simulink model "radio_enlace"  (R2017a)
settings: Solver=ode45  StartTime=0.0  StopTime=Inf  RelTol=1e-3  EnableMultiTasking=on
libraries: dsparch4 x5, commfilt2 x3, commdigbbndpm3 x2, commsink2 x1, simulink x1, dspstat3 x1, commrflib2 x1, commchan3 x1, commrandsrc2 x1
settings Model: Creator=ampl  LastModifiedBy=rubem
settings DataIOCC: LimitDataPoints=on  SaveFormat=Array
settings OptimizationCC: LifeSpan=inf
settings DebuggingCC: UnderspecifiedInitializationDetection=Classic  MergeDetectMultiDrivingBlocksExec=none  SolverPrmCheckMsg=warning  SFUnexpectedBacktrackingDiag=warning  SFNoUnconditionalDefaultTransitionDiag=warning  SFExecutionAtInitializationDiag=none
settings HardwareCC: ProdBitPerPointer=32  ProdBitPerSizeT=32  ProdBitPerPtrDiffT=32  ProdLargestAtomicFloat=None  ProdIntDivRoundTo=Undefined  ProdEndianess=Unspecified  ProdWordSize=32  ProdHWDeviceType=32-bit Generic
settings ModelReferenceCC: PropagateSignalLabelsOutOfModel=off
settings GRTTargetCC: TargetLangStandard=C89/C90 (ANSI)  GeneratePreprocessorConditionals=Disable all
settings ConfigComp: CovMetricSettings=dw  CovHtmlReporting=on  CovSaveCumulativeToWorkspaceVar=on  CovSaveSingleToWorkspaceVar=on  CovExternalEMLEnable=off

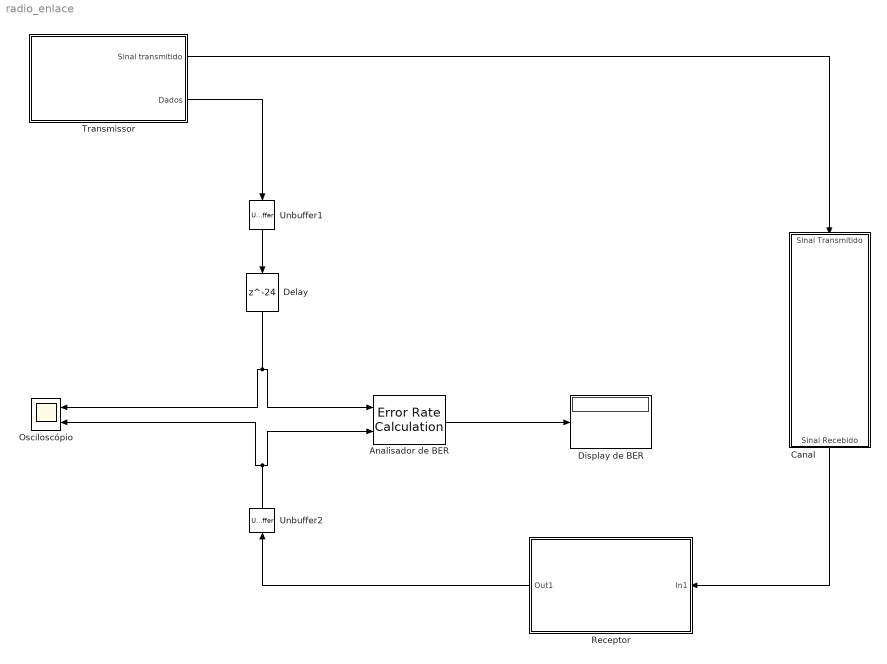
== system radio_enlace ==
  Analisador de BER : commsink2/Error Rate Calculation  N=0  st_delay=1e3  cp_mode=Entire frame  subframe=[]  PMode=Port  WsName=ErrorVec  RsMode2=off  stop=off  numErr=100  maxBits=1e6
  Canal : Subsystem
  Delay : Delay  DelayLength=24
  Display de BER : Display
  Osciloscópio : Scope  NumInputPorts=2
  Receptor : Subsystem
  Transmissor : Subsystem
  Unbuffer1 : Unbuffer
  Unbuffer2 : Unbuffer
  wires:
  Analisador de BER/1 -> Display de BER/1
  Unbuffer1/1 -> Delay/1
  Transmissor/2(Dados) -> Unbuffer1/1
  Transmissor/1(Sinal transmitido) -> Canal/1(Sinal Transmitido)
  Canal/1(Sinal Recebido) -> Receptor/1(In1)
  Receptor/1(Out1) -> Unbuffer2/1
  Unbuffer2/1 -> Osciloscópio/2, Analisador de BER/2
  Delay/1 -> Osciloscópio/1, Analisador de BER/1

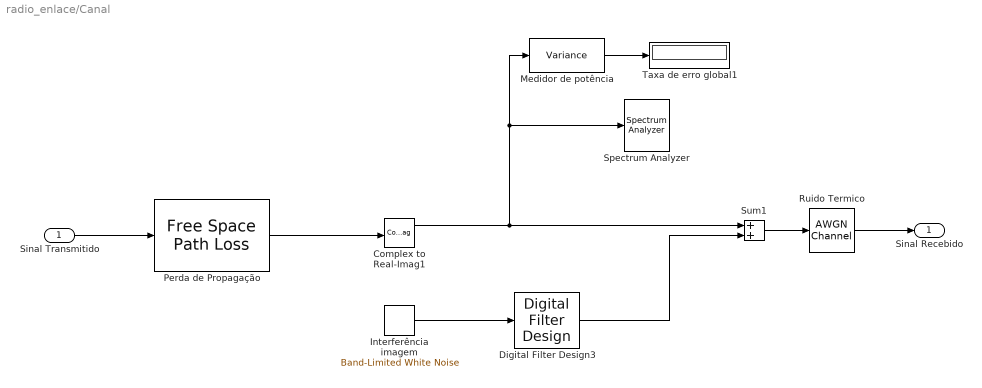
== system radio_enlace/Canal ==
  Sinal Transmitido : Inport
  Complex to Real-Imag1 : ComplexToRealImag
  Digital Filter Design3 : dsparch4/Digital Filter Design  mwdsp_browser_bugfix_var=off
  Interferência imagem : simulink/Sources/Band-Limited White Noise  Cov=[0.0001]  Ts=1/4000e6  seed=[23341]
  Medidor de potência : dspstat3/Variance  run=on  reset_popup=None  InputProcessing=Columns as channels (frame based)  directionMode=Each column  dimension=1  roiEnable=off  roiType=Rectangles  roiPortion=Entire ROI  roiOutput=Individual statistics for each ROI  roiFlag=off  roundingMode=Floor  overflowMode=off
      settings: SourceProductName=DSP System Toolbox
  Perda de Propagação : commrflib2/Free Space Path Loss  mode=Decibels  dB=0  d=0.100  fc=1920
      settings: SourceProductName=Communications System Toolbox  SourceProductBaseCode=CM
  Ruido Termico : commchan3/AWGN Channel  InputProcessing=Columns as channels (frame based)  seed=67  noiseMode="Signal to noise ratio  (Eb/No)"  EbNodB=5  EsNodB=10  SNRdB=10  bitsPerSym=2  Ps=0.000625  Tsym=1/5e6  variance=1
  Spectrum Analyzer : SpectrumAnalyzer
  Sum1 : Sum  Inputs=+|+
  Taxa de erro global1 : Display
  Sinal Recebido : Outport
  wires:
  Sum1/1 -> Ruido Termico/1
  Ruido Termico/1 -> Sinal Recebido/1
  Complex to Real-Imag1/1 -> Spectrum Analyzer/1, Medidor de potência/1, Sum1/1
  Perda de Propagação/1 -> Complex to Real-Imag1/1
  Interferência imagem/1 -> Digital Filter Design3/1
  Medidor de potência/1 -> Taxa de erro global1/1
  Digital Filter Design3/1 -> Sum1/2
  Sinal Transmitido/1 -> Perda de Propagação/1

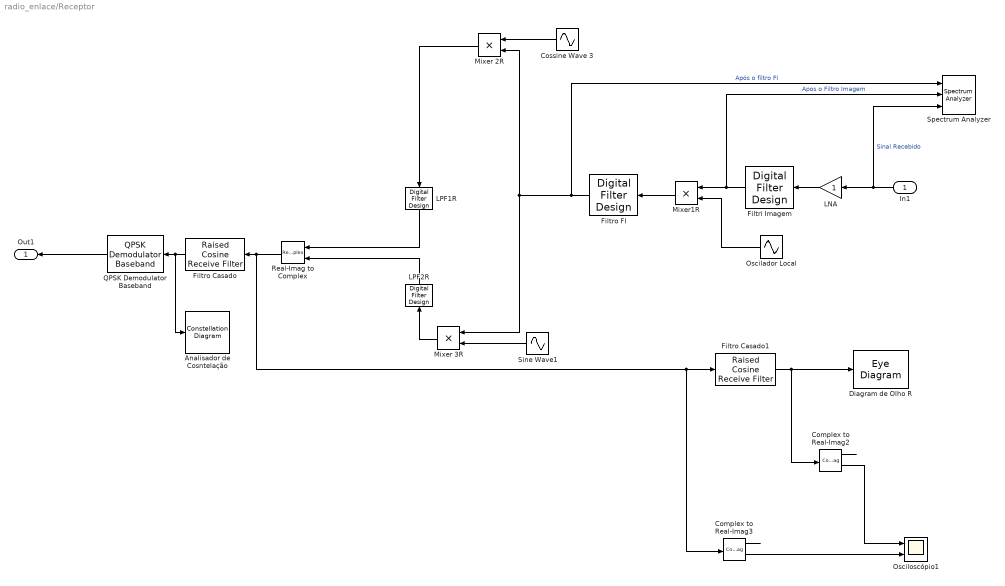
== system radio_enlace/Receptor ==
  In1 : Inport
  Analisador de Cosntelação : ConstellationDiagram
  Complex to Real-Imag2 : ComplexToRealImag
  Complex to Real-Imag3 : ComplexToRealImag
  Cossine Wave 3 : Sin  Frequency=2*pi*(70e6)  Phase=pi/2  Samples=4  SampleTime=1/4000e6
  Diagram de Olho R : EyeDiagram  Tag=EyeDiagram
  Filtri Imagem : dsparch4/Digital Filter Design  mwdsp_browser_bugfix_var=off
  Filtro Casado : commfilt2/Raised Cosine Receive Filter  filtType=Square root  R=0.5  filtSpan=10  N=800  downFactor=800  downOffset=60  filterGain=4  InputProcessing=Columns as channels (frame based)  RateOptions=Allow multirate processing  framing=Mute  checkCoeff=off  variableName=rcRxFilt  currentFiltSpan=10  D=5  inputOffset=0  sampMode=Mute  saveAsFlag=0  rateMode=Downsampling  checkGain=Normalized  launchFVT=on  roundingMode=Floor  overflowMode=off  coeffDataTypeStr=Inherit: Same word length as input  coeffMin=[]  coeffMax=[]  coeffLastDataTypeStr=Inherit: Same word length as input  accumDataTypeStr=Inherit: Same as product output  accumLastDataTypeStr=Inherit: Same as product output  outputDataTypeStr=Inherit: Same as accumulator  outputMin=[]  outputMax=[]  outputLastDataTypeStr=Inherit: Same as accumulator
  Filtro Casado1 : commfilt2/Raised Cosine Receive Filter  filtType=Square root  R=0.5  filtSpan=10  N=800  downFactor=1  downOffset=0  filterGain=4  InputProcessing=Columns as channels (frame based)  RateOptions=Allow multirate processing  framing=Mute  checkCoeff=off  variableName=rcRxFilt1  currentFiltSpan=10  D=5  inputOffset=0  sampMode=Mute  saveAsFlag=0  rateMode=Downsampling  checkGain=Normalized  launchFVT=on  roundingMode=Floor  overflowMode=off  coeffDataTypeStr=Inherit: Same word length as input  coeffMin=[]  coeffMax=[]  coeffLastDataTypeStr=Inherit: Same word length as input  accumDataTypeStr=Inherit: Same as product output  accumLastDataTypeStr=Inherit: Same as product output  outputDataTypeStr=Inherit: Same as accumulator  outputMin=[]  outputMax=[]  outputLastDataTypeStr=Inherit: Same as accumulator
  Filtro FI : dsparch4/Digital Filter Design  mwdsp_browser_bugfix_var=off
  LNA : Gain
  LPF1R : dsparch4/Digital Filter Design  mwdsp_browser_bugfix_var=off
  LPF2R : dsparch4/Digital Filter Design  mwdsp_browser_bugfix_var=off
  Mixer 2R : Product  RndMeth=Zero
  Mixer 3R : Product  RndMeth=Zero
  Mixer1R : Product  RndMeth=Zero
  Oscilador Local : Sin  Frequency=2*pi*(930e6)  Phase=pi/2  Samples=4  SampleTime=1/4000e6
  Osciloscópio1 : Scope  NumInputPorts=2
  QPSK Demodulator Baseband : commdigbbndpm3/QPSK Demodulator Baseband  OutType=Bit  DecType=Hard decision  VarSource=Dialog  Variance=1  Dec=Gray  Ph=pi/4  outDtype1=Inherit via internal rule  outDtype2=Inherit via internal rule  derotateFactorWordLen=16  derotateFactorDataTypeStr=Inherit: Same word length as input  derotateFactorLastDataTypeStr=Inherit: Same word length as input
  Real-Imag to Complex : RealImagToComplex
  Sine Wave1 : Sin  Frequency=2*pi*(70e6)  Phase=pi  Samples=4  SampleTime=1/4000e6
  Spectrum Analyzer : SpectrumAnalyzer  NumInputPorts=3
  Out1 : Outport
  wires:
  QPSK Demodulator Baseband/1 -> Out1/1
  Sine Wave1/1 -> Mixer 3R/2
  LPF2R/1 -> Real-Imag to Complex/2
  Filtro FI/1 -> Spectrum Analyzer/1, Mixer 3R/1, Mixer 2R/2  "Após o filtro FI"
  LNA/1 -> Filtri Imagem/1
  Oscilador Local/1 -> Mixer1R/2
  Filtro Casado/1 -> Analisador de Cosntelação/1, QPSK Demodulator Baseband/1
  Complex to Real-Imag2/2 -> Osciloscópio1/1
  Complex to Real-Imag3/2 -> Osciloscópio1/2
  Filtro Casado1/1 -> Complex to Real-Imag2/1, Diagram de Olho R/1
  Mixer 3R/1 -> LPF2R/1
  Mixer1R/1 -> Filtro FI/1
  LPF1R/1 -> Real-Imag to Complex/1
  Mixer 2R/1 -> LPF1R/1
  Filtri Imagem/1 -> Spectrum Analyzer/2, Mixer1R/1  "Apos o Filtro Imagem"
  Real-Imag to Complex/1 -> Filtro Casado1/1, Complex to Real-Imag3/1, Filtro Casado/1
  Cossine Wave 3/1 -> Mixer 2R/1
  In1/1 -> Spectrum Analyzer/3, LNA/1  "Sinal Recebido"
  Complex to Real-Imag2/1 -> ?
  Complex to Real-Imag3/1 -> ?

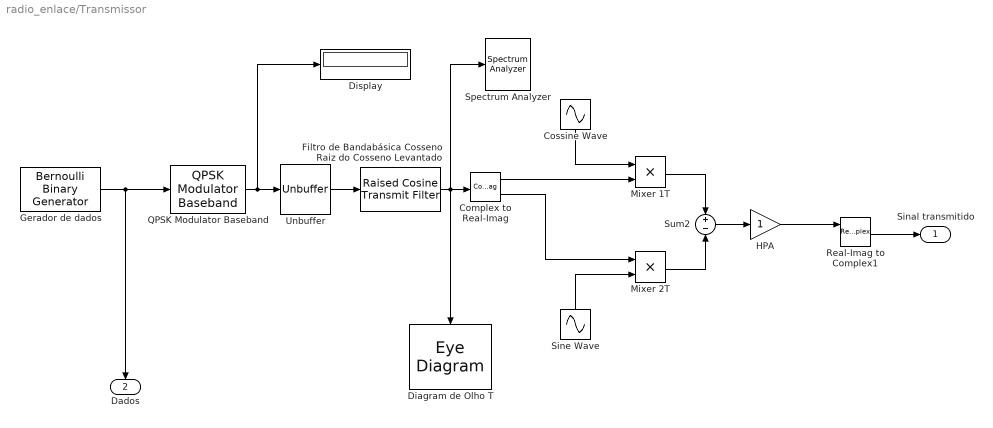
== system radio_enlace/Transmissor ==
  Complex to Real-Imag : ComplexToRealImag
  "Cossine Wave " : Sin  Frequency=2*pi*(1000e6)  Phase=pi/2  Samples=4  SampleTime=1/4000e6
  Diagram de Olho T : EyeDiagram  Tag=EyeDiagram
  Display : Display
  Filtro de Bandabásica Cosseno Raiz do Cosseno Levantado : commfilt2/Raised Cosine Transmit Filter  filtType=Square root  R=0  filtSpan=10  N=800  filterGain=1  InputProcessing=Columns as channels (frame based)  RateOptions=Allow multirate processing  framing=Mute  checkCoeff=off  variableName=rcTxFilt  checkGain=Normalized  sampMode=Mute  saveAsFlag=0  currentFiltSpan=10  D=5  launchFVT=on  roundingMode=Floor  overflowMode=off  coeffDataTypeStr=Inherit: Same word length as input  coeffMin=[]  coeffMax=[]  coeffLastDataTypeStr=Inherit: Same word length as input  outputDataTypeStr=Inherit: Same as accumulator  outputMin=[]  outputMax=[]  outputLastDataTypeStr=Inherit: Same as accumulator
  Gerador de dados : commrandsrc2/Bernoulli Binary Generator  P=0.5  seed=61  Ts=1/10e6  frameBased=on  sampPerFrame=2  orient=off  outDataType=double
  HPA : Gain
  Mixer 1T : Product  RndMeth=Zero
  Mixer 2T : Product  RndMeth=Zero
  QPSK Modulator Baseband : commdigbbndpm3/QPSK Modulator Baseband  InType=Bit  Enc=Gray  Ph=pi/4  outDtype=double  outWordLen=16  outUDDataType=sfix(16)  outFracLenMode=Best precision  outFracLen=15  outDataTypeStr=double  outLastDataTypeStr=double
  Real-Imag to Complex1 : RealImagToComplex
  Sine Wave : Sin  Frequency=2*pi*(1000e6)  Samples=4  SampleTime=1/4000e6
  Spectrum Analyzer : SpectrumAnalyzer
  Sum2 : Sum  Inputs=+|-
  Unbuffer : Unbuffer
  Sinal transmitido : Outport
  Dados : Outport  Port=2
  wires:
  Gerador de dados/1 -> Dados/1, QPSK Modulator Baseband/1
  Unbuffer/1 -> Filtro de Bandabásica Cosseno Raiz do Cosseno Levantado/1
  "Cossine Wave "/1 -> Mixer 1T/1
  Complex to Real-Imag/1 -> Mixer 1T/2
  Mixer 2T/1 -> Sum2/2
  Filtro de Bandabásica Cosseno Raiz do Cosseno Levantado/1 -> Spectrum Analyzer/1, Complex to Real-Imag/1, Diagram de Olho T/1
  Mixer 1T/1 -> Sum2/1
  Complex to Real-Imag/2 -> Mixer 2T/1
  HPA/1 -> Real-Imag to Complex1/1
  Sine Wave/1 -> Mixer 2T/2
  Sum2/1 -> HPA/1
  Real-Imag to Complex1/1 -> Sinal transmitido/1
  QPSK Modulator Baseband/1 -> Display/1, Unbuffer/1
